simulink model "Scissor_Lift_4_Hydraulic_Actuator"  (R2016a)
settings: Solver=ode23t  StartTime=0.0  StopTime=10.0  MaxStep=1e-2  RelTol=1e-3  AbsTol=1e-4
PostLoadFcn:
  | warning off Simulink:Engine:OutputNotConnected
  | warning off mech2:compiler:topologyAnalysis:DanglingBlock
undefined symbols (not defined in the file): Local, Scissor_Lift_Param, X, Y, Z
libraries: sm_lib x48, Scissor_Parts_Lib x21, fl_lib x8, nesl_utility x7, sh_lib x4
(part 1 of 2)
Description:
  | Copyright 2014-2016 The MathWorks, Inc.
settings Model: Creator=smiller  LastModifiedBy=smiller
settings DataIOCC: LimitDataPoints=on  SaveFormat=Array  SignalLoggingSaveFormat=ModelDataLogs
settings OptimizationCC: ExpressionDepthLimit=2147483647
settings DebuggingCC: UnderspecifiedInitializationDetection=Classic  MergeDetectMultiDrivingBlocksExec=none  SolverPrmCheckMsg=warning  FcnCallInpInsideContextMsg=EnableAllAsWarning  AllowSymbolicDim=off  StateNameClashWarn=warning
settings HardwareCC: ProdBitPerPointer=32  ProdLargestAtomicFloat=None  ProdIntDivRoundTo=Undefined  ProdEndianess=Unspecified  ProdWordSize=32  ProdHWDeviceType=32-bit Generic
settings ModelReferenceCC: PropagateSignalLabelsOutOfModel=off
settings ConfigComp: CovModelRefEnable=Off  CovSFcnEnable=off
settings SimscapeCC: SimscapeLogType=all
settings ConfigurationSet: Description=SimMechanics 2G
settings ExplorerConfigSet: InternalSimMechanicsExplorerSettings="<ExplorerConfiguration><canonicalview>default</canonicalview><TilePanel><TileInfo><Tiles Columns=\"1\" Count=\"1\" Rows=\"1\"><Column Left=\"2\" Weight=\"1\"/><Column Left=\"398\"/><Row Top=\"2\" Weight=\"1\"/><Row Top=\"485\"/><Tile Height=\"1\" Width=\"1\" X=\"0\" Y=\"0\"/></Tiles></TileInfo><SceneInfo><SceneViewer><BGColor><R>0.60000002384185791</R><G>0.60000002384185791</G><B>0.60000002384185791</B></BGColor><Camera><Position><X>7.1151910018991291</X><Y>-6.9387533499588399</Y><Z>5.7460715877417217</Z></Position><Center><X>1.3999999761581421</X><Y>0</Y><Z>2.540661096572876</Z></Center><Up><X>-0.23055989473784222</X><Y>0.24511291789662082</Y><Z>0.94168030266045166</Z></Up><Left>-1.6691677093505861</Left><Right>1.6691677093505861</Right><Bottom>-3.5760457992553714</Bottom><Top>3.5760457992553714</Top></Camera></SceneViewer></SceneInfo></TilePanel></ExplorerConfiguration>"

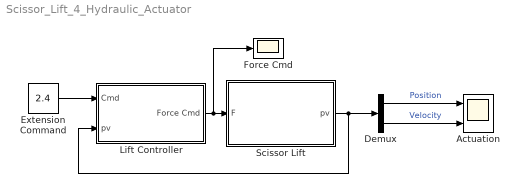
== system Scissor_Lift_4_Hydraulic_Actuator ==
  Actuation : Scope  NumInputPorts=2
  Demux : Demux  Outputs=2
  Extension Command : Constant  Value=2.4
  Force Cmd : Scope
  Lift Controller : Subsystem
  Scissor Lift : Subsystem
      mask Display:
      | image(imread('Scissor_Lift_3Stage_IMAGE.jpg'));
      | port_label('input',1,'F');
      | port_label('output',1,'pv');
  wires:
  Extension Command/1 -> Lift Controller/1(Cmd)
  Lift Controller/1(Force Cmd) -> Scissor Lift/1(F), Force Cmd/1
  Scissor Lift/1(pv) -> Lift Controller/2(pv), Demux/1
  Demux/1 -> Actuation/1  "Position"
  Demux/2 -> Actuation/2  "Velocity"

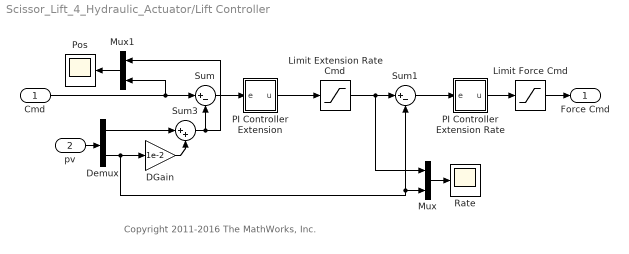
== system Scissor_Lift_4_Hydraulic_Actuator/Lift Controller ==
  note: Copyright 2011-2016 The MathWorks, Inc.
  Cmd : Inport
  pv : Inport  Port=2
  DGain : Gain  Gain=1e-2
  Demux : Demux  Outputs=2
  Limit Extension Rate Cmd : Saturate
  Limit Force Cmd : Saturate  UpperLimit=1e6  LowerLimit=-1e6
  Mux : Mux  Inputs=2
  Mux1 : Mux  Inputs=2
  PI Controller Extension : Subsystem
      mask Display:
      | plot([0 1],[0 0]);
      | plot([1 2],[0 1]);
      | plot([2 3],[1 1]);
      | disp('P I');
  PI Controller Extension Rate : Subsystem
      mask Display:
      | plot([0 1],[0 0]);
      | plot([1 2],[0 1]);
      | plot([2 3],[1 1]);
      | disp('P I');
  Pos : Scope
  Rate : Scope
  Sum : Sum  Inputs=|+-
  Sum1 : Sum  Inputs=|+-
  Sum3 : Sum  Inputs=|++
  Force Cmd : Outport
  wires:
  PI Controller Extension Rate/1(u) -> Limit Force Cmd/1
  PI Controller Extension/1(u) -> Limit Extension Rate Cmd/1
  Sum1/1 -> PI Controller Extension Rate/1(e)
  Limit Extension Rate Cmd/1 -> Sum1/1, Mux/1
  DGain/1 -> Sum3/2
  Sum3/1 -> Sum/2, Mux1/1
  Cmd/1 -> Sum/1, Mux1/2
  Sum/1 -> PI Controller Extension/1(e)
  Demux/2 -> DGain/1, Sum1/2, Mux/2
  Limit Force Cmd/1 -> Force Cmd/1
  Demux/1 -> Sum3/1
  pv/1 -> Demux/1
  Mux/1 -> Rate/1
  Mux1/1 -> Pos/1

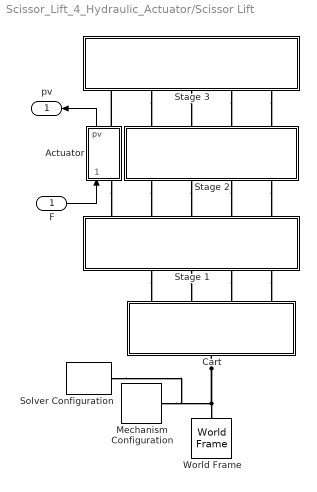
== system Scissor_Lift_4_Hydraulic_Actuator/Scissor Lift ==
  F : Inport
  Actuator : Subsystem
  Cart : Subsystem
  Mechanism Configuration : sm_lib/Utilities/Mechanism Configuration  UniformGravity=Constant  GravityVector=[0 0 -9.81]  GravityUnits=m/s^2  LinearizationDelta=0.001
  Solver Configuration : nesl_utility/Solver Configuration  PhysicalDomain=network_engine_domain  SubClassName=solver  LeftPortType=input  RightPortType=generic  Accelerate=off  Tones=[]  Harmonics=[]  SimulateNoise=off  Profile=off  UseLocalSampling=off  EnableSwitchedLinearOptims=on  FrequencyDomain=off  UseCCode=off  RelTol=0.001  AbsTol=1e-06  MinStep=1e-09  ToWorkspace=off  RevertToSquareIcSolve=off  NumHomotopyIterations=100  PhasorMode=off  PhasorModeNumHarmonics=1  OverrideAbsTol=off  DoDC=off  ResidualTolerance=1e-9  UseLocalSolver=off  LocalSolverChoice=NE_BACKWARD_EULER_ADVANCER  LocalSolverSampleTime=.001  DoFixedCost=off  MaxNonlinIter=3  MaxModeIter=2  LinearAlgebra=Sparse  DelaysMemoryBudget=1024  AutomaticFiltering=on  FilteringTimeConstant=0.001
  Stage 1 : Subsystem
  Stage 2 : Subsystem
  Stage 3 : Subsystem
  World Frame : sm_lib/Frames and Transforms/World Frame
  pv : Outport
  wires:
  Actuator/1(pv) -> pv/1
  F/1 -> Actuator/1(Vsig)
  connections:
  Actuator/LConn1 -- Stage 1/LConn1
  Actuator/RConn1 -- Stage 3/RConn1
  Cart/LConn1 -- Mechanism Configuration/RConn1 -- Solver Configuration/RConn1 -- World Frame/RConn1
  Stage 1/RConn2 -- Cart/RConn1
  Stage 1/RConn3 -- Cart/RConn2
  Stage 1/RConn4 -- Cart/RConn3
  Stage 1/RConn5 -- Cart/RConn4
  Stage 2/RConn1 -- Stage 1/LConn2
  Stage 2/RConn2 -- Stage 1/LConn3
  Stage 2/RConn3 -- Stage 1/LConn4
  Stage 2/RConn4 -- Stage 1/LConn5
  Stage 3/RConn2 -- Stage 2/LConn1
  Stage 3/RConn3 -- Stage 2/LConn2
  Stage 3/RConn4 -- Stage 2/LConn3
  Stage 3/RConn5 -- Stage 2/LConn4

== system Scissor_Lift_4_Hydraulic_Actuator/Lift Controller/PI Controller Extension ==
  e : Inport
  Integral Gain : Gain  Gain=100  SaturateOnIntegerOverflow=on  OutDataTypeStr=Inherit: Same as input  ParamDataTypeStr=Inherit: Same as input
  Integrator : Integrator  LimitOutput=on  UpperSaturationLimit=1  LowerSaturationLimit=-1
  Proportional Gain : Gain  Gain=8e2  SaturateOnIntegerOverflow=on  OutDataTypeStr=Inherit: Same as input  ParamDataTypeStr=Inherit: Same as input
  Sum : Sum  Inputs=++|  SaturateOnIntegerOverflow=on  InputSameDT=on  OutDataTypeStr=Inherit: Same as first input
  u : Outport  InitialOutput=0
  wires:
  Sum/1 -> u/1
  e/1 -> Integral Gain/1, Proportional Gain/1
  Integrator/1 -> Sum/2
  Proportional Gain/1 -> Sum/1
  Integral Gain/1 -> Integrator/1

== system Scissor_Lift_4_Hydraulic_Actuator/Lift Controller/PI Controller Extension Rate ==
  e : Inport
  Integral Gain : Gain  Gain=100  SaturateOnIntegerOverflow=on  OutDataTypeStr=Inherit: Same as input  ParamDataTypeStr=Inherit: Same as input
  Integrator : Integrator  LimitOutput=on  UpperSaturationLimit=1e6  LowerSaturationLimit=-1e6
  Proportional Gain : Gain  Gain=3e6  SaturateOnIntegerOverflow=on  OutDataTypeStr=Inherit: Same as input  ParamDataTypeStr=Inherit: Same as input
  Sum : Sum  Inputs=++|  SaturateOnIntegerOverflow=on  InputSameDT=on  OutDataTypeStr=Inherit: Same as first input
  u : Outport  InitialOutput=0
  wires:
  Integral Gain/1 -> Integrator/1
  Proportional Gain/1 -> Sum/1
  Integrator/1 -> Sum/2
  e/1 -> Proportional Gain/1, Integral Gain/1
  Sum/1 -> u/1

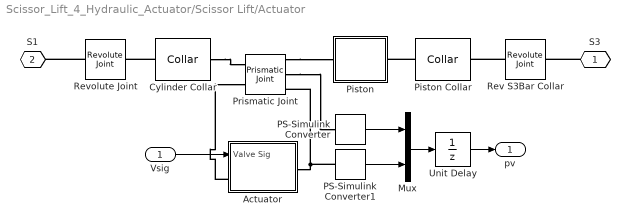
== system Scissor_Lift_4_Hydraulic_Actuator/Scissor Lift/Actuator ==
  Vsig : Inport
  Actuator : Subsystem
  Cylinder Collar : Scissor_Parts_Lib/Collar  collar_length=Scissor_Lift_Param.Actuator.Collar.Length  collar_radius=Scissor_Lift_Param.Actuator.Collar.Radius  cylinder_length=Scissor_Lift_Param.Actuator.Cylinder.Length  cylinder_radius=Scissor_Lift_Param.Actuator.Cylinder.Radius  cylinder_ori=Local +Z  material_density=Scissor_Lift_Param.Actuator.Collar.Density  material_color=Scissor_Lift_Param.Actuator.Collar.Color  material_opacity=Scissor_Lift_Param.Actuator.Collar.Opacity
  Mux : Mux  Inputs=2
  PS-Simulink Converter : nesl_utility/PS-Simulink Converter  PhysicalDomain=network_engine_domain  SubClassName=ps_output  LeftPortType=input  RightPortType=output  PseudoPeriodic=off  Frequencies=[]  Unit=1  AffineConversion=off
  PS-Simulink Converter1 : nesl_utility/PS-Simulink Converter  PhysicalDomain=network_engine_domain  SubClassName=ps_output  LeftPortType=input  RightPortType=output  PseudoPeriodic=off  Frequencies=[]  Unit=1  AffineConversion=off
  Piston : Subsystem
      mask Display:
      | image(imread('Piston_Shaft_IMAGE.jpg'));
      | port_label('RConn',1,'P');
      | port_label('LConn',1,'R');
  Piston Collar : Scissor_Parts_Lib/Collar  collar_length=Scissor_Lift_Param.Actuator.Collar.Length  collar_radius=Scissor_Lift_Param.Actuator.Collar.Radius  cylinder_length=Scissor_Lift_Param.Actuator.Piston_Seat.Length  cylinder_radius=Scissor_Lift_Param.Actuator.Piston_Seat.Radius  cylinder_ori=Local -Z  material_density=Scissor_Lift_Param.Actuator.Collar.Density  material_color=Scissor_Lift_Param.Actuator.Collar.Color  material_opacity=Scissor_Lift_Param.Actuator.Collar.Opacity
  Prismatic Joint : sm_lib/Joints/Prismatic Joint  SenseConstraintForce=off  SenseConstraintForceX=off  SenseConstraintForceY=off  SenseConstraintForceZ=off  SenseConstraintTorque=off  SenseConstraintTorqueX=off  SenseConstraintTorqueY=off  SenseConstraintTorqueZ=off  SenseTotalForce=off  SenseTotalForceX=off  SenseTotalForceY=off  SenseTotalForceZ=off  SenseTotalTorque=off  SenseTotalTorqueX=off  SenseTotalTorqueY=off  SenseTotalTorqueZ=off  CompositeWrenchDir=FollowerOnBase  CompositeWrenchFrame=BaseFrame  EquilibriumPosition=Scissor_Lift_Param.Actuator.Spring.Equilibrium_Position*0  EquilibriumPositionUnits=cm  SpringStiffness=Scissor_Lift_Param.Actuator.Spring.Stiffness*0  SpringStiffnessUnits=N/m  DampingCoefficient=Scissor_Lift_Param.Actuator.Spring.Damping*0+2000  DampingCoefficientUnits=N/(m/s)  TorqueActuationMode=InputTorque  MotionActuationMode=ComputedMotion  SensePosition=on  SenseVelocity=on  SenseAcceleration=off  SenseTorqueForce=off  PositionTargetSpecify=off  PositionTargetPriority=High  PositionTargetValue=0  PositionTargetValueUnits=m  VelocityTargetSpecify=off  VelocityTargetPriority=High  VelocityTargetValue=0  VelocityTargetValueUnits=m/s
  Rev S3Bar Collar : sm_lib/Joints/Revolute Joint  SenseConstraintForce=off  SenseConstraintForceX=off  SenseConstraintForceY=off  SenseConstraintForceZ=off  SenseConstraintTorque=off  SenseConstraintTorqueX=off  SenseConstraintTorqueY=off  SenseConstraintTorqueZ=off  SenseTotalForce=off  SenseTotalForceX=off  SenseTotalForceY=off  SenseTotalForceZ=off  SenseTotalTorque=off  SenseTotalTorqueX=off  SenseTotalTorqueY=off  SenseTotalTorqueZ=off  CompositeWrenchDir=FollowerOnBase  CompositeWrenchFrame=BaseFrame  EquilibriumPosition=0  EquilibriumPositionUnits=rad  SpringStiffness=0  SpringStiffnessUnits=N*m/rad  DampingCoefficient=0  DampingCoefficientUnits=N*m/(rad/s)  TorqueActuationMode=NoTorque  MotionActuationMode=ComputedMotion  SensePosition=off  SenseVelocity=off  SenseAcceleration=off  SenseTorqueForce=off  PositionTargetSpecify=off  PositionTargetPriority=High  PositionTargetValue=0  PositionTargetValueUnits=rad  VelocityTargetSpecify=off  VelocityTargetPriority=High  VelocityTargetValue=0  VelocityTargetValueUnits=rad/s
  Revolute Joint : sm_lib/Joints/Revolute Joint  SenseConstraintForce=off  SenseConstraintForceX=off  SenseConstraintForceY=off  SenseConstraintForceZ=off  SenseConstraintTorque=off  SenseConstraintTorqueX=off  SenseConstraintTorqueY=off  SenseConstraintTorqueZ=off  SenseTotalForce=off  SenseTotalForceX=off  SenseTotalForceY=off  SenseTotalForceZ=off  SenseTotalTorque=off  SenseTotalTorqueX=off  SenseTotalTorqueY=off  SenseTotalTorqueZ=off  CompositeWrenchDir=FollowerOnBase  CompositeWrenchFrame=BaseFrame  EquilibriumPosition=0  EquilibriumPositionUnits=rad  SpringStiffness=0  SpringStiffnessUnits=N*m/rad  DampingCoefficient=0  DampingCoefficientUnits=N*m/(rad/s)  TorqueActuationMode=NoTorque  MotionActuationMode=ComputedMotion  SensePosition=off  SenseVelocity=off  SenseAcceleration=off  SenseTorqueForce=off  PositionTargetSpecify=off  PositionTargetPriority=High  PositionTargetValue=0  PositionTargetValueUnits=rad  VelocityTargetSpecify=off  VelocityTargetPriority=High  VelocityTargetValue=0  VelocityTargetValueUnits=rad/s
  Unit Delay : UnitDelay  InitialCondition=1.755  SampleTime=0.01
  S3 : PMIOPort  Port=1  Side=Right
  S1 : PMIOPort  Port=2  Side=Left
  pv : Outport
  wires:
  Vsig/1 -> Actuator/1(Valve Sig)
  PS-Simulink Converter/1 -> Mux/1
  PS-Simulink Converter1/1 -> Mux/2
  Mux/1 -> Unit Delay/1
  Unit Delay/1 -> pv/1
  connections:
  Cylinder Collar/LConn1 -- Revolute Joint/RConn1
  Cylinder Collar/RConn1 -- Prismatic Joint/LConn1
  Prismatic Joint/RConn1 -- Piston/RConn1
  Piston Collar/RConn1 -- Piston/LConn1
  Rev S3Bar Collar/RConn1 -- Piston Collar/LConn1
  S3/RConn1 -- Rev S3Bar Collar/LConn1
  Revolute Joint/LConn1 -- S1/RConn1
  Prismatic Joint/RConn2 -- PS-Simulink Converter/LConn1
  Actuator/LConn1 -- Prismatic Joint/LConn2
  PS-Simulink Converter1/LConn1 -- Prismatic Joint/RConn3 -- Actuator/RConn1

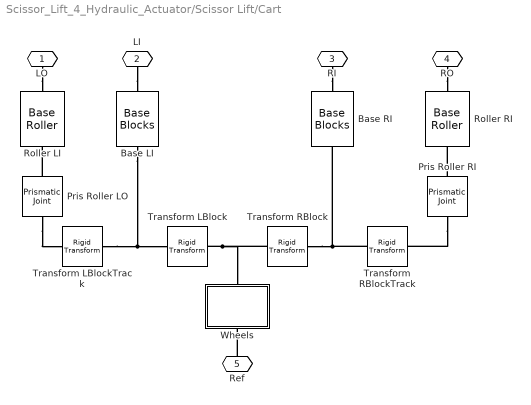
== system Scissor_Lift_4_Hydraulic_Actuator/Scissor Lift/Cart ==
  Base LI : Scissor_Parts_Lib/Base Blocks  block_length=Scissor_Lift_Param.Base_Block.Length  block_width=Scissor_Lift_Param.Base_Block.Width  block_height=Scissor_Lift_Param.Base_Block.Height  shaft_radius=Scissor_Lift_Param.Roller.Shaft_Radius  shaft_length=Scissor_Lift_Param.Roller.Shaft_Length  material_density=Scissor_Lift_Param.Base_Block.Density  material_color=Scissor_Lift_Param.Base_Block.Color  material_opacity=Scissor_Lift_Param.Base_Block.Opacity
  Base RI : Scissor_Parts_Lib/Base Blocks  block_length=Scissor_Lift_Param.Base_Block.Length  block_width=Scissor_Lift_Param.Base_Block.Width  block_height=Scissor_Lift_Param.Base_Block.Height  shaft_radius=Scissor_Lift_Param.Roller.Shaft_Radius  shaft_length=Scissor_Lift_Param.Roller.Shaft_Length  material_density=Scissor_Lift_Param.Base_Block.Density  material_color=Scissor_Lift_Param.Base_Block.Color  material_opacity=Scissor_Lift_Param.Base_Block.Opacity
  Pris Roller LO : sm_lib/Joints/Prismatic Joint  SenseConstraintForce=off  SenseConstraintForceX=off  SenseConstraintForceY=off  SenseConstraintForceZ=off  SenseConstraintTorque=off  SenseConstraintTorqueX=off  SenseConstraintTorqueY=off  SenseConstraintTorqueZ=off  SenseTotalForce=off  SenseTotalForceX=off  SenseTotalForceY=off  SenseTotalForceZ=off  SenseTotalTorque=off  SenseTotalTorqueX=off  SenseTotalTorqueY=off  SenseTotalTorqueZ=off  CompositeWrenchDir=FollowerOnBase  CompositeWrenchFrame=BaseFrame  EquilibriumPosition=0  EquilibriumPositionUnits=m  SpringStiffness=0  SpringStiffnessUnits=N/m  DampingCoefficient=0  DampingCoefficientUnits=N/(m/s)  TorqueActuationMode=NoTorque  MotionActuationMode=ComputedMotion  SensePosition=off  SenseVelocity=off  SenseAcceleration=off  SenseTorqueForce=off  PositionTargetSpecify=on  PositionTargetPriority=High  PositionTargetValue=Scissor_Lift_Param.Roller.Init_Pos_Target  PositionTargetValueUnits=cm  VelocityTargetSpecify=off  VelocityTargetPriority=High  VelocityTargetValue=0  VelocityTargetValueUnits=m/s
  Pris Roller RI : sm_lib/Joints/Prismatic Joint  SenseConstraintForce=off  SenseConstraintForceX=off  SenseConstraintForceY=off  SenseConstraintForceZ=off  SenseConstraintTorque=off  SenseConstraintTorqueX=off  SenseConstraintTorqueY=off  SenseConstraintTorqueZ=off  SenseTotalForce=off  SenseTotalForceX=off  SenseTotalForceY=off  SenseTotalForceZ=off  SenseTotalTorque=off  SenseTotalTorqueX=off  SenseTotalTorqueY=off  SenseTotalTorqueZ=off  CompositeWrenchDir=FollowerOnBase  CompositeWrenchFrame=BaseFrame  EquilibriumPosition=0  EquilibriumPositionUnits=m  SpringStiffness=0  SpringStiffnessUnits=N/m  DampingCoefficient=0  DampingCoefficientUnits=N/(m/s)  TorqueActuationMode=NoTorque  MotionActuationMode=ComputedMotion  SensePosition=off  SenseVelocity=off  SenseAcceleration=off  SenseTorqueForce=off  PositionTargetSpecify=off  PositionTargetPriority=High  PositionTargetValue=0  PositionTargetValueUnits=m  VelocityTargetSpecify=off  VelocityTargetPriority=High  VelocityTargetValue=0  VelocityTargetValueUnits=m/s
  Roller LI : Scissor_Parts_Lib/Base Roller  roller_length=Scissor_Lift_Param.Roller.Roller_Length  roller_radius=Scissor_Lift_Param.Roller.Roller_Radius  shaft_length=Scissor_Lift_Param.Roller.Shaft_Length  shaft_radius=Scissor_Lift_Param.Roller.Shaft_Radius  material_density=Scissor_Lift_Param.Roller.Density  material_color=Scissor_Lift_Param.Roller.Color  material_opacity=Scissor_Lift_Param.Roller.Opacity
  Roller RI : Scissor_Parts_Lib/Base Roller  roller_length=Scissor_Lift_Param.Roller.Roller_Length  roller_radius=Scissor_Lift_Param.Roller.Roller_Radius  shaft_length=Scissor_Lift_Param.Roller.Shaft_Length  shaft_radius=Scissor_Lift_Param.Roller.Shaft_Radius  material_density=Scissor_Lift_Param.Roller.Density  material_color=Scissor_Lift_Param.Roller.Color  material_opacity=Scissor_Lift_Param.Roller.Opacity
  Transform LBlock : sm_lib/Frames and Transforms/Rigid Transform  TranslationMethod=Cartesian  TranslationLengthUnit=cm  TranslationStandardAxis=+Y  TranslationStandardOffset=Scissor_Lift_Param.Cart.Platform.Height/2  TranslationCartesianOffset=[20 0 Scissor_Lift_Param.Link_Separation.Outer_Outer/2-Scissor_Lift_Param.Link_Separation.Outer_Inner]  TranslationROffset=0  TranslationROffsetUnits=m  TranslationZOffset=0  TranslationZOffsetUnits=m  TranslationThetaOffset=0  TranslationThetaOffsetUnits=deg  RotationMethod=None  RotationAngleUnits=deg  RotationStandardAxis=+X  RotationAngle=90  RotationArbitraryAxis=[0 0 1]  FollAlignAxisA=+X  BaseAlignAxisA=+Y  FollAlignAxisB=+Y  BaseAlignAxisB=+Z  RotationSequenceAxes=FollowerAxes  RotationSequence=XYX  RotationSequenceAngles=[0 0 0]  RotationSequenceAnglesUnits=deg  RotationMatrix=[1 0 0; 0 1 0; 0 0 1]
  Transform LBlockTrack : sm_lib/Frames and Transforms/Rigid Transform  TranslationMethod=StandardAxis  TranslationLengthUnit=cm  TranslationStandardAxis=+Z  TranslationStandardOffset=Scissor_Lift_Param.Link_Separation.Outer_Inner  TranslationCartesianOffset=[0 0 0]  TranslationROffset=0  TranslationROffsetUnits=m  TranslationZOffset=0  TranslationZOffsetUnits=m  TranslationThetaOffset=0  TranslationThetaOffsetUnits=deg  RotationMethod=StandardAxis  RotationAngleUnits=deg  RotationStandardAxis=+Y  RotationAngle=90  RotationArbitraryAxis=[0 0 1]  FollAlignAxisA=+X  BaseAlignAxisA=+Y  FollAlignAxisB=+Y  BaseAlignAxisB=+Z  RotationSequenceAxes=FollowerAxes  RotationSequence=XYX  RotationSequenceAngles=[0 0 0]  RotationSequenceAnglesUnits=deg  RotationMatrix=[1 0 0; 0 1 0; 0 0 1]
  Transform RBlock : sm_lib/Frames and Transforms/Rigid Transform  TranslationMethod=Cartesian  TranslationLengthUnit=cm  TranslationStandardAxis=+Y  TranslationStandardOffset=Scissor_Lift_Param.Cart.Platform.Height/2  TranslationCartesianOffset=[20 0 -Scissor_Lift_Param.Link_Separation.Outer_Outer/2+Scissor_Lift_Param.Link_Separation.Outer_Inner]  TranslationROffset=0  TranslationROffsetUnits=m  TranslationZOffset=0  TranslationZOffsetUnits=m  TranslationThetaOffset=0  TranslationThetaOffsetUnits=deg  RotationMethod=None  RotationAngleUnits=deg  RotationStandardAxis=+X  RotationAngle=90  RotationArbitraryAxis=[0 0 1]  FollAlignAxisA=+X  BaseAlignAxisA=+Y  FollAlignAxisB=+Y  BaseAlignAxisB=+Z  RotationSequenceAxes=FollowerAxes  RotationSequence=XYX  RotationSequenceAngles=[0 0 0]  RotationSequenceAnglesUnits=deg  RotationMatrix=[1 0 0; 0 1 0; 0 0 1]
  Transform RBlockTrack : sm_lib/Frames and Transforms/Rigid Transform  TranslationMethod=StandardAxis  TranslationLengthUnit=cm  TranslationStandardAxis=-Z  TranslationStandardOffset=Scissor_Lift_Param.Link_Separation.Outer_Inner  TranslationCartesianOffset=[0 0 0]  TranslationROffset=0  TranslationROffsetUnits=m  TranslationZOffset=0  TranslationZOffsetUnits=m  TranslationThetaOffset=0  TranslationThetaOffsetUnits=deg  RotationMethod=StandardAxis  RotationAngleUnits=deg  RotationStandardAxis=+Y  RotationAngle=90  RotationArbitraryAxis=[0 0 1]  FollAlignAxisA=+X  BaseAlignAxisA=+Y  FollAlignAxisB=+Y  BaseAlignAxisB=+Z  RotationSequenceAxes=FollowerAxes  RotationSequence=XYX  RotationSequenceAngles=[0 0 0]  RotationSequenceAnglesUnits=deg  RotationMatrix=[1 0 0; 0 1 0; 0 0 1]
  Wheels : Subsystem
  LO : PMIOPort  Port=1  Side=Right
  LI : PMIOPort  Port=2  Side=Right
  RI : PMIOPort  Port=3  Side=Right
  RO : PMIOPort  Port=4  Side=Right
  Ref : PMIOPort  Port=5  Side=Left
  connections:
  Pris Roller LO/LConn1 -- Transform LBlockTrack/RConn1
  Pris Roller LO/RConn1 -- Roller LI/LConn1
  Transform LBlockTrack/LConn1 -- Base LI/LConn1 -- Transform LBlock/RConn1
  Transform RBlockTrack/LConn1 -- Base RI/LConn1 -- Transform RBlock/RConn1
  Pris Roller RI/LConn1 -- Transform RBlockTrack/RConn1
  Pris Roller RI/RConn1 -- Roller RI/LConn1
  Ref/RConn1 -- Wheels/LConn1
  LO/RConn1 -- Roller LI/RConn1
  LI/RConn1 -- Base LI/RConn1
  RO/RConn1 -- Roller RI/RConn1
  RI/RConn1 -- Base RI/RConn1
  Transform LBlock/LConn1 -- Wheels/RConn1 -- Transform RBlock/LConn1

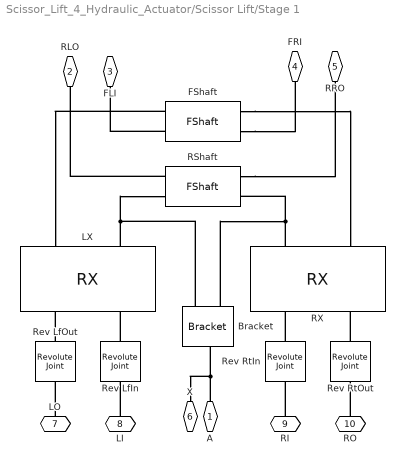
== system Scissor_Lift_4_Hydraulic_Actuator/Scissor Lift/Stage 1 ==
  Bracket : Scissor_Parts_Lib/Bracket  fl_w=Scissor_Lift_Param.Actuator.Bracket.Flange.Width  fl_h=Scissor_Lift_Param.Actuator.Bracket.Flange.Height  T=Scissor_Lift_Param.Actuator.Bracket.Flange.Thickness  W=Scissor_Lift_Param.Actuator.Bracket.Flange.Offset  flupdown=Down  flfrontrear=Rear  fl_density=Scissor_Lift_Param.Actuator.Bracket.Flange.Density  fl_clr=Scissor_Lift_Param.Actuator.Bracket.Flange.Color  fl_opc=Scissor_Lift_Param.Actuator.Bracket.Flange.Opacity  shaft_length=Scissor_Lift_Param.Link_Separation.Outer_Outer-Scissor_Lift_Param.Link_Separation.Outer_Inner*2  shaft_radius=Scissor_Lift_Param.Actuator.Bracket.Shaft.Radius  shaft_density=Scissor_Lift_Param.Actuator.Bracket.Shaft.Density  shaft_color=Scissor_Lift_Param.Actuator.Bracket.Shaft.Color  shaft_opacity=Scissor_Lift_Param.Actuator.Bracket.Shaft.Opacity
  FShaft : Scissor_Parts_Lib/FShaft  sep_outer_outer=Scissor_Lift_Param.Link_Separation.Outer_Outer  sep_outer_inner=Scissor_Lift_Param.Link_Separation.Outer_Inner  shaft_radius=Scissor_Lift_Param.Trans_Shaft.Radius  shaft_density=Scissor_Lift_Param.Trans_Shaft.Density  shaft_color=Scissor_Lift_Param.Trans_Shaft.Color  shaft_opacity=Scissor_Lift_Param.Trans_Shaft.Opacity
  LX : Scissor_Parts_Lib/RX  link_length=Scissor_Lift_Param.Link.Length  link_width=Scissor_Lift_Param.Link.Width  link_thickness=Scissor_Lift_Param.Link.Thickness  link_hole_radius=Scissor_Lift_Param.Link.Hole_Radius  link_density=Scissor_Lift_Param.Link.Density  link_color=Scissor_Lift_Param.Link.Color  link_opacity=Scissor_Lift_Param.Link.Opacity  shaft_length=Scissor_Lift_Param.Link_Separation.Outer_Inner  shaft_radius=Scissor_Lift_Param.Link_Pin.Radius  shaft_density=Scissor_Lift_Param.Link_Pin.Density  shaft_color=Scissor_Lift_Param.Link_Pin.Color  shaft_opacity=Scissor_Lift_Param.Link_Pin.Opacity  leftright=Left  imgfile=Crossbar_RX_IMAGE.jpg  L1Port=OU  L2Port=IU  R1Port=OL  R2Port=IL
  RShaft : Scissor_Parts_Lib/FShaft  sep_outer_outer=Scissor_Lift_Param.Link_Separation.Outer_Outer  sep_outer_inner=Scissor_Lift_Param.Link_Separation.Outer_Inner  shaft_radius=Scissor_Lift_Param.Trans_Shaft.Radius  shaft_density=Scissor_Lift_Param.Trans_Shaft.Density  shaft_color=Scissor_Lift_Param.Trans_Shaft.Color  shaft_opacity=Scissor_Lift_Param.Trans_Shaft.Opacity
  RX : Scissor_Parts_Lib/RX  link_length=Scissor_Lift_Param.Link.Length  link_width=Scissor_Lift_Param.Link.Width  link_thickness=Scissor_Lift_Param.Link.Thickness  link_hole_radius=Scissor_Lift_Param.Link.Hole_Radius  link_density=Scissor_Lift_Param.Link.Density  link_color=Scissor_Lift_Param.Link.Color  link_opacity=Scissor_Lift_Param.Link.Opacity  shaft_length=Scissor_Lift_Param.Link_Separation.Outer_Inner  shaft_radius=Scissor_Lift_Param.Link_Pin.Radius  shaft_density=Scissor_Lift_Param.Link_Pin.Density  shaft_color=Scissor_Lift_Param.Link_Pin.Color  shaft_opacity=Scissor_Lift_Param.Link_Pin.Opacity  leftright=Right  imgfile=Crossbar_RX_IMAGE.jpg  L1Port=OU  L2Port=IU  R1Port=OL  R2Port=IL
  Rev LfIn : sm_lib/Joints/Revolute Joint  SenseConstraintForce=off  SenseConstraintForceX=off  SenseConstraintForceY=off  SenseConstraintForceZ=off  SenseConstraintTorque=off  SenseConstraintTorqueX=off  SenseConstraintTorqueY=off  SenseConstraintTorqueZ=off  SenseTotalForce=off  SenseTotalForceX=off  SenseTotalForceY=off  SenseTotalForceZ=off  SenseTotalTorque=off  SenseTotalTorqueX=off  SenseTotalTorqueY=off  SenseTotalTorqueZ=off  CompositeWrenchDir=FollowerOnBase  CompositeWrenchFrame=BaseFrame  EquilibriumPosition=0  EquilibriumPositionUnits=rad  SpringStiffness=0  SpringStiffnessUnits=N*m/rad  DampingCoefficient=0  DampingCoefficientUnits=N*m/(rad/s)  TorqueActuationMode=NoTorque  MotionActuationMode=ComputedMotion  SensePosition=off  SenseVelocity=off  SenseAcceleration=off  SenseTorqueForce=off  PositionTargetSpecify=off  PositionTargetPriority=Low  PositionTargetValue=0  PositionTargetValueUnits=deg  VelocityTargetSpecify=off  VelocityTargetPriority=High  VelocityTargetValue=0  VelocityTargetValueUnits=rad/s
  Rev LfOut : sm_lib/Joints/Revolute Joint  SenseConstraintForce=off  SenseConstraintForceX=off  SenseConstraintForceY=off  SenseConstraintForceZ=off  SenseConstraintTorque=off  SenseConstraintTorqueX=off  SenseConstraintTorqueY=off  SenseConstraintTorqueZ=off  SenseTotalForce=off  SenseTotalForceX=off  SenseTotalForceY=off  SenseTotalForceZ=off  SenseTotalTorque=off  SenseTotalTorqueX=off  SenseTotalTorqueY=off  SenseTotalTorqueZ=off  CompositeWrenchDir=FollowerOnBase  CompositeWrenchFrame=BaseFrame  EquilibriumPosition=0  EquilibriumPositionUnits=rad  SpringStiffness=0  SpringStiffnessUnits=N*m/rad  DampingCoefficient=0  DampingCoefficientUnits=N*m/(rad/s)  TorqueActuationMode=NoTorque  MotionActuationMode=ComputedMotion  SensePosition=off  SenseVelocity=off  SenseAcceleration=off  SenseTorqueForce=off  PositionTargetSpecify=on  PositionTargetPriority=Low  PositionTargetValue=Scissor_Lift_Param.Crossbar.Init_Angle_Target  PositionTargetValueUnits=deg  VelocityTargetSpecify=off  VelocityTargetPriority=High  VelocityTargetValue=0  VelocityTargetValueUnits=rad/s
  Rev RtIn : sm_lib/Joints/Revolute Joint  SenseConstraintForce=off  SenseConstraintForceX=off  SenseConstraintForceY=off  SenseConstraintForceZ=off  SenseConstraintTorque=off  SenseConstraintTorqueX=off  SenseConstraintTorqueY=off  SenseConstraintTorqueZ=off  SenseTotalForce=off  SenseTotalForceX=off  SenseTotalForceY=off  SenseTotalForceZ=off  SenseTotalTorque=off  SenseTotalTorqueX=off  SenseTotalTorqueY=off  SenseTotalTorqueZ=off  CompositeWrenchDir=FollowerOnBase  CompositeWrenchFrame=BaseFrame  EquilibriumPosition=0  EquilibriumPositionUnits=rad  SpringStiffness=0  SpringStiffnessUnits=N*m/rad  DampingCoefficient=0  DampingCoefficientUnits=N*m/(rad/s)  TorqueActuationMode=NoTorque  MotionActuationMode=ComputedMotion  SensePosition=off  SenseVelocity=off  SenseAcceleration=off  SenseTorqueForce=off  PositionTargetSpecify=off  PositionTargetPriority=Low  PositionTargetValue=0  PositionTargetValueUnits=deg  VelocityTargetSpecify=off  VelocityTargetPriority=High  VelocityTargetValue=0  VelocityTargetValueUnits=rad/s
  Rev RtOut : sm_lib/Joints/Revolute Joint  SenseConstraintForce=off  SenseConstraintForceX=off  SenseConstraintForceY=off  SenseConstraintForceZ=off  SenseConstraintTorque=off  SenseConstraintTorqueX=off  SenseConstraintTorqueY=off  SenseConstraintTorqueZ=off  SenseTotalForce=off  SenseTotalForceX=off  SenseTotalForceY=off  SenseTotalForceZ=off  SenseTotalTorque=off  SenseTotalTorqueX=off  SenseTotalTorqueY=off  SenseTotalTorqueZ=off  CompositeWrenchDir=FollowerOnBase  CompositeWrenchFrame=BaseFrame  EquilibriumPosition=0  EquilibriumPositionUnits=rad  SpringStiffness=0  SpringStiffnessUnits=N*m/rad  DampingCoefficient=0  DampingCoefficientUnits=N*m/(rad/s)  TorqueActuationMode=NoTorque  MotionActuationMode=ComputedMotion  SensePosition=off  SenseVelocity=off  SenseAcceleration=off  SenseTorqueForce=off  PositionTargetSpecify=off  PositionTargetPriority=Low  PositionTargetValue=0  PositionTargetValueUnits=deg  VelocityTargetSpecify=off  VelocityTargetPriority=High  VelocityTargetValue=0  VelocityTargetValueUnits=rad/s
  A : PMIOPort  Port=1  Side=Left
  RLO : PMIOPort  Port=2  Side=Left
  FLI : PMIOPort  Port=3  Side=Left
  FRI : PMIOPort  Port=4  Side=Left
  RRO : PMIOPort  Port=5  Side=Left
  X : PMIOPort  Port=6  Side=Right
  LO : PMIOPort  Port=7  Side=Right
  LI : PMIOPort  Port=8  Side=Right
  RI : PMIOPort  Port=9  Side=Right
  RO : PMIOPort  Port=10  Side=Right
  connections:
  FShaft/LConn1 -- LX/LConn1
  FShaft/LConn2 -- FLI/RConn1
  FShaft/RConn1 -- RX/LConn2
  FShaft/RConn2 -- FRI/RConn1
  LX/LConn2 -- RShaft/LConn2 -- Bracket/RConn1
  Rev LfOut/RConn1 -- LX/RConn1
  Rev LfIn/RConn1 -- LX/RConn2
  RShaft/LConn1 -- RLO/RConn1
  RShaft/RConn1 -- RRO/RConn1
  RX/LConn1 -- RShaft/RConn2 -- Bracket/RConn2
  Rev RtIn/RConn1 -- RX/RConn1
  Rev RtOut/RConn1 -- RX/RConn2
  LI/RConn1 -- Rev LfIn/LConn1
  LO/RConn1 -- Rev LfOut/LConn1
  RI/RConn1 -- Rev RtIn/LConn1
  RO/RConn1 -- Rev RtOut/LConn1
  Bracket/LConn1 -- X/RConn1 -- A/RConn1

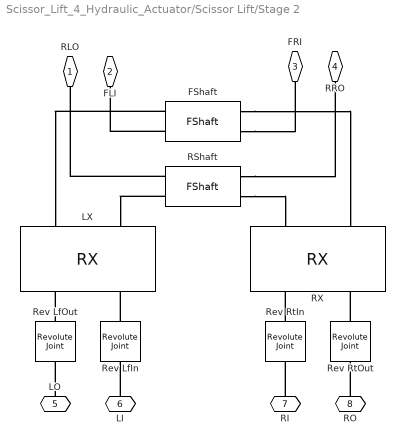
== system Scissor_Lift_4_Hydraulic_Actuator/Scissor Lift/Stage 2 ==
  FShaft : Scissor_Parts_Lib/FShaft  sep_outer_outer=Scissor_Lift_Param.Link_Separation.Outer_Outer  sep_outer_inner=Scissor_Lift_Param.Link_Separation.Outer_Inner  shaft_radius=Scissor_Lift_Param.Trans_Shaft.Radius  shaft_density=Scissor_Lift_Param.Trans_Shaft.Density  shaft_color=Scissor_Lift_Param.Trans_Shaft.Color  shaft_opacity=Scissor_Lift_Param.Trans_Shaft.Opacity
  LX : Scissor_Parts_Lib/RX  link_length=Scissor_Lift_Param.Link.Length  link_width=Scissor_Lift_Param.Link.Width  link_thickness=Scissor_Lift_Param.Link.Thickness  link_hole_radius=Scissor_Lift_Param.Link.Hole_Radius  link_density=Scissor_Lift_Param.Link.Density  link_color=Scissor_Lift_Param.Link.Color  link_opacity=Scissor_Lift_Param.Link.Opacity  shaft_length=Scissor_Lift_Param.Link_Separation.Outer_Inner  shaft_radius=Scissor_Lift_Param.Link_Pin.Radius  shaft_density=Scissor_Lift_Param.Link_Pin.Density  shaft_color=Scissor_Lift_Param.Link_Pin.Color  shaft_opacity=Scissor_Lift_Param.Link_Pin.Opacity  leftright=Left  imgfile=Crossbar_RX_IMAGE.jpg  L1Port=OU  L2Port=IU  R1Port=OL  R2Port=IL
  RShaft : Scissor_Parts_Lib/FShaft  sep_outer_outer=Scissor_Lift_Param.Link_Separation.Outer_Outer  sep_outer_inner=Scissor_Lift_Param.Link_Separation.Outer_Inner  shaft_radius=Scissor_Lift_Param.Trans_Shaft.Radius  shaft_density=Scissor_Lift_Param.Trans_Shaft.Density  shaft_color=Scissor_Lift_Param.Trans_Shaft.Color  shaft_opacity=Scissor_Lift_Param.Trans_Shaft.Opacity
  RX : Scissor_Parts_Lib/RX  link_length=Scissor_Lift_Param.Link.Length  link_width=Scissor_Lift_Param.Link.Width  link_thickness=Scissor_Lift_Param.Link.Thickness  link_hole_radius=Scissor_Lift_Param.Link.Hole_Radius  link_density=Scissor_Lift_Param.Link.Density  link_color=Scissor_Lift_Param.Link.Color  link_opacity=Scissor_Lift_Param.Link.Opacity  shaft_length=Scissor_Lift_Param.Link_Separation.Outer_Inner  shaft_radius=Scissor_Lift_Param.Link_Pin.Radius  shaft_density=Scissor_Lift_Param.Link_Pin.Density  shaft_color=Scissor_Lift_Param.Link_Pin.Color  shaft_opacity=Scissor_Lift_Param.Link_Pin.Opacity  leftright=Right  imgfile=Crossbar_RX_IMAGE.jpg  L1Port=OU  L2Port=IU  R1Port=OL  R2Port=IL
  Rev LfIn : sm_lib/Joints/Revolute Joint  SenseConstraintForce=off  SenseConstraintForceX=off  SenseConstraintForceY=off  SenseConstraintForceZ=off  SenseConstraintTorque=off  SenseConstraintTorqueX=off  SenseConstraintTorqueY=off  SenseConstraintTorqueZ=off  SenseTotalForce=off  SenseTotalForceX=off  SenseTotalForceY=off  SenseTotalForceZ=off  SenseTotalTorque=off  SenseTotalTorqueX=off  SenseTotalTorqueY=off  SenseTotalTorqueZ=off  CompositeWrenchDir=FollowerOnBase  CompositeWrenchFrame=BaseFrame  EquilibriumPosition=0  EquilibriumPositionUnits=rad  SpringStiffness=0  SpringStiffnessUnits=N*m/rad  DampingCoefficient=0  DampingCoefficientUnits=N*m/(rad/s)  TorqueActuationMode=NoTorque  MotionActuationMode=ComputedMotion  SensePosition=off  SenseVelocity=off  SenseAcceleration=off  SenseTorqueForce=off  PositionTargetSpecify=off  PositionTargetPriority=Low  PositionTargetValue=0  PositionTargetValueUnits=deg  VelocityTargetSpecify=off  VelocityTargetPriority=High  VelocityTargetValue=0  VelocityTargetValueUnits=rad/s
  Rev LfOut : sm_lib/Joints/Revolute Joint  SenseConstraintForce=off  SenseConstraintForceX=off  SenseConstraintForceY=off  SenseConstraintForceZ=off  SenseConstraintTorque=off  SenseConstraintTorqueX=off  SenseConstraintTorqueY=off  SenseConstraintTorqueZ=off  SenseTotalForce=off  SenseTotalForceX=off  SenseTotalForceY=off  SenseTotalForceZ=off  SenseTotalTorque=off  SenseTotalTorqueX=off  SenseTotalTorqueY=off  SenseTotalTorqueZ=off  CompositeWrenchDir=FollowerOnBase  CompositeWrenchFrame=BaseFrame  EquilibriumPosition=0  EquilibriumPositionUnits=rad  SpringStiffness=0  SpringStiffnessUnits=N*m/rad  DampingCoefficient=0  DampingCoefficientUnits=N*m/(rad/s)  TorqueActuationMode=NoTorque  MotionActuationMode=ComputedMotion  SensePosition=off  SenseVelocity=off  SenseAcceleration=off  SenseTorqueForce=off  PositionTargetSpecify=on  PositionTargetPriority=Low  PositionTargetValue=2*Scissor_Lift_Param.Crossbar.Init_Angle_Target  PositionTargetValueUnits=deg  VelocityTargetSpecify=off  VelocityTargetPriority=High  VelocityTargetValue=0  VelocityTargetValueUnits=rad/s
  Rev RtIn : sm_lib/Joints/Revolute Joint  SenseConstraintForce=off  SenseConstraintForceX=off  SenseConstraintForceY=off  SenseConstraintForceZ=off  SenseConstraintTorque=off  SenseConstraintTorqueX=off  SenseConstraintTorqueY=off  SenseConstraintTorqueZ=off  SenseTotalForce=off  SenseTotalForceX=off  SenseTotalForceY=off  SenseTotalForceZ=off  SenseTotalTorque=off  SenseTotalTorqueX=off  SenseTotalTorqueY=off  SenseTotalTorqueZ=off  CompositeWrenchDir=FollowerOnBase  CompositeWrenchFrame=BaseFrame  EquilibriumPosition=0  EquilibriumPositionUnits=rad  SpringStiffness=0  SpringStiffnessUnits=N*m/rad  DampingCoefficient=0  DampingCoefficientUnits=N*m/(rad/s)  TorqueActuationMode=NoTorque  MotionActuationMode=ComputedMotion  SensePosition=off  SenseVelocity=off  SenseAcceleration=off  SenseTorqueForce=off  PositionTargetSpecify=off  PositionTargetPriority=Low  PositionTargetValue=0  PositionTargetValueUnits=deg  VelocityTargetSpecify=off  VelocityTargetPriority=High  VelocityTargetValue=0  VelocityTargetValueUnits=rad/s
  Rev RtOut : sm_lib/Joints/Revolute Joint  SenseConstraintForce=off  SenseConstraintForceX=off  SenseConstraintForceY=off  SenseConstraintForceZ=off  SenseConstraintTorque=off  SenseConstraintTorqueX=off  SenseConstraintTorqueY=off  SenseConstraintTorqueZ=off  SenseTotalForce=off  SenseTotalForceX=off  SenseTotalForceY=off  SenseTotalForceZ=off  SenseTotalTorque=off  SenseTotalTorqueX=off  SenseTotalTorqueY=off  SenseTotalTorqueZ=off  CompositeWrenchDir=FollowerOnBase  CompositeWrenchFrame=BaseFrame  EquilibriumPosition=0  EquilibriumPositionUnits=rad  SpringStiffness=0  SpringStiffnessUnits=N*m/rad  DampingCoefficient=0  DampingCoefficientUnits=N*m/(rad/s)  TorqueActuationMode=NoTorque  MotionActuationMode=ComputedMotion  SensePosition=off  SenseVelocity=off  SenseAcceleration=off  SenseTorqueForce=off  PositionTargetSpecify=off  PositionTargetPriority=Low  PositionTargetValue=0  PositionTargetValueUnits=deg  VelocityTargetSpecify=off  VelocityTargetPriority=High  VelocityTargetValue=0  VelocityTargetValueUnits=rad/s
  RLO : PMIOPort  Port=1  Side=Left
  FLI : PMIOPort  Port=2  Side=Left
  FRI : PMIOPort  Port=3  Side=Left
  RRO : PMIOPort  Port=4  Side=Left
  LO : PMIOPort  Port=5  Side=Right
  LI : PMIOPort  Port=6  Side=Right
  RI : PMIOPort  Port=7  Side=Right
  RO : PMIOPort  Port=8  Side=Right
  connections:
  RO/RConn1 -- Rev RtOut/LConn1
  RI/RConn1 -- Rev RtIn/LConn1
  LO/RConn1 -- Rev LfOut/LConn1
  LI/RConn1 -- Rev LfIn/LConn1
  Rev RtOut/RConn1 -- RX/RConn2
  Rev RtIn/RConn1 -- RX/RConn1
  RShaft/RConn2 -- RX/LConn1
  RShaft/RConn1 -- RRO/RConn1
  RShaft/LConn1 -- RLO/RConn1
  Rev LfIn/RConn1 -- LX/RConn2
  Rev LfOut/RConn1 -- LX/RConn1
  RShaft/LConn2 -- LX/LConn2
  FShaft/RConn2 -- FRI/RConn1
  FShaft/RConn1 -- RX/LConn2
  FShaft/LConn2 -- FLI/RConn1
  FShaft/LConn1 -- LX/LConn1

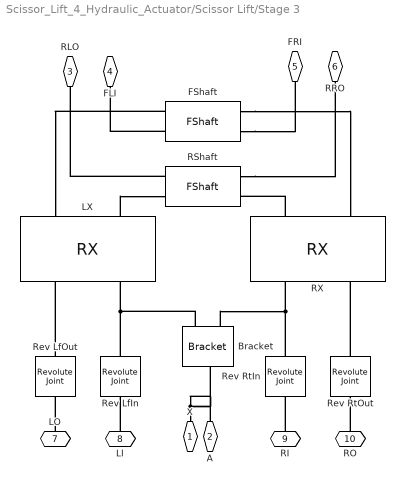
== system Scissor_Lift_4_Hydraulic_Actuator/Scissor Lift/Stage 3 ==
  Bracket : Scissor_Parts_Lib/Bracket  fl_w=Scissor_Lift_Param.Actuator.Bracket.Flange.Width  fl_h=Scissor_Lift_Param.Actuator.Bracket.Flange.Height  T=Scissor_Lift_Param.Actuator.Bracket.Flange.Thickness  W=Scissor_Lift_Param.Actuator.Bracket.Flange.Offset  flupdown=Up  flfrontrear=Front  fl_density=Scissor_Lift_Param.Actuator.Bracket.Flange.Density  fl_clr=Scissor_Lift_Param.Actuator.Bracket.Flange.Color  fl_opc=Scissor_Lift_Param.Actuator.Bracket.Flange.Opacity  shaft_length=Scissor_Lift_Param.Link_Separation.Outer_Outer-Scissor_Lift_Param.Link_Separation.Outer_Inner*2  shaft_radius=Scissor_Lift_Param.Actuator.Bracket.Shaft.Radius  shaft_density=Scissor_Lift_Param.Actuator.Bracket.Shaft.Density  shaft_color=Scissor_Lift_Param.Actuator.Bracket.Shaft.Color  shaft_opacity=Scissor_Lift_Param.Actuator.Bracket.Shaft.Opacity
  FShaft : Scissor_Parts_Lib/FShaft  sep_outer_outer=Scissor_Lift_Param.Link_Separation.Outer_Outer  sep_outer_inner=Scissor_Lift_Param.Link_Separation.Outer_Inner  shaft_radius=Scissor_Lift_Param.Trans_Shaft.Radius  shaft_density=Scissor_Lift_Param.Trans_Shaft.Density  shaft_color=Scissor_Lift_Param.Trans_Shaft.Color  shaft_opacity=Scissor_Lift_Param.Trans_Shaft.Opacity
  LX : Scissor_Parts_Lib/RX  link_length=Scissor_Lift_Param.Link.Length  link_width=Scissor_Lift_Param.Link.Width  link_thickness=Scissor_Lift_Param.Link.Thickness  link_hole_radius=Scissor_Lift_Param.Link.Hole_Radius  link_density=Scissor_Lift_Param.Link.Density  link_color=Scissor_Lift_Param.Link.Color  link_opacity=Scissor_Lift_Param.Link.Opacity  shaft_length=Scissor_Lift_Param.Link_Separation.Outer_Inner  shaft_radius=Scissor_Lift_Param.Link_Pin.Radius  shaft_density=Scissor_Lift_Param.Link_Pin.Density  shaft_color=Scissor_Lift_Param.Link_Pin.Color  shaft_opacity=Scissor_Lift_Param.Link_Pin.Opacity  leftright=Left  imgfile=Crossbar_RX_IMAGE.jpg  L1Port=OU  L2Port=IU  R1Port=OL  R2Port=IL
  RShaft : Scissor_Parts_Lib/FShaft  sep_outer_outer=Scissor_Lift_Param.Link_Separation.Outer_Outer  sep_outer_inner=Scissor_Lift_Param.Link_Separation.Outer_Inner  shaft_radius=Scissor_Lift_Param.Trans_Shaft.Radius  shaft_density=Scissor_Lift_Param.Trans_Shaft.Density  shaft_color=Scissor_Lift_Param.Trans_Shaft.Color  shaft_opacity=Scissor_Lift_Param.Trans_Shaft.Opacity
  RX : Scissor_Parts_Lib/RX  link_length=Scissor_Lift_Param.Link.Length  link_width=Scissor_Lift_Param.Link.Width  link_thickness=Scissor_Lift_Param.Link.Thickness  link_hole_radius=Scissor_Lift_Param.Link.Hole_Radius  link_density=Scissor_Lift_Param.Link.Density  link_color=Scissor_Lift_Param.Link.Color  link_opacity=Scissor_Lift_Param.Link.Opacity  shaft_length=Scissor_Lift_Param.Link_Separation.Outer_Inner  shaft_radius=Scissor_Lift_Param.Link_Pin.Radius  shaft_density=Scissor_Lift_Param.Link_Pin.Density  shaft_color=Scissor_Lift_Param.Link_Pin.Color  shaft_opacity=Scissor_Lift_Param.Link_Pin.Opacity  leftright=Right  imgfile=Crossbar_RX_IMAGE.jpg  L1Port=OU  L2Port=IU  R1Port=OL  R2Port=IL
  Rev LfIn : sm_lib/Joints/Revolute Joint  SenseConstraintForce=off  SenseConstraintForceX=off  SenseConstraintForceY=off  SenseConstraintForceZ=off  SenseConstraintTorque=off  SenseConstraintTorqueX=off  SenseConstraintTorqueY=off  SenseConstraintTorqueZ=off  SenseTotalForce=off  SenseTotalForceX=off  SenseTotalForceY=off  SenseTotalForceZ=off  SenseTotalTorque=off  SenseTotalTorqueX=off  SenseTotalTorqueY=off  SenseTotalTorqueZ=off  CompositeWrenchDir=FollowerOnBase  CompositeWrenchFrame=BaseFrame  EquilibriumPosition=0  EquilibriumPositionUnits=rad  SpringStiffness=0  SpringStiffnessUnits=N*m/rad  DampingCoefficient=0  DampingCoefficientUnits=N*m/(rad/s)  TorqueActuationMode=NoTorque  MotionActuationMode=ComputedMotion  SensePosition=off  SenseVelocity=off  SenseAcceleration=off  SenseTorqueForce=off  PositionTargetSpecify=off  PositionTargetPriority=Low  PositionTargetValue=0  PositionTargetValueUnits=deg  VelocityTargetSpecify=off  VelocityTargetPriority=High  VelocityTargetValue=0  VelocityTargetValueUnits=rad/s
  Rev LfOut : sm_lib/Joints/Revolute Joint  SenseConstraintForce=off  SenseConstraintForceX=off  SenseConstraintForceY=off  SenseConstraintForceZ=off  SenseConstraintTorque=off  SenseConstraintTorqueX=off  SenseConstraintTorqueY=off  SenseConstraintTorqueZ=off  SenseTotalForce=off  SenseTotalForceX=off  SenseTotalForceY=off  SenseTotalForceZ=off  SenseTotalTorque=off  SenseTotalTorqueX=off  SenseTotalTorqueY=off  SenseTotalTorqueZ=off  CompositeWrenchDir=FollowerOnBase  CompositeWrenchFrame=BaseFrame  EquilibriumPosition=0  EquilibriumPositionUnits=rad  SpringStiffness=0  SpringStiffnessUnits=N*m/rad  DampingCoefficient=0  DampingCoefficientUnits=N*m/(rad/s)  TorqueActuationMode=NoTorque  MotionActuationMode=ComputedMotion  SensePosition=off  SenseVelocity=off  SenseAcceleration=off  SenseTorqueForce=off  PositionTargetSpecify=on  PositionTargetPriority=Low  PositionTargetValue=2*Scissor_Lift_Param.Crossbar.Init_Angle_Target  PositionTargetValueUnits=deg  VelocityTargetSpecify=off  VelocityTargetPriority=High  VelocityTargetValue=0  VelocityTargetValueUnits=rad/s
  Rev RtIn : sm_lib/Joints/Revolute Joint  SenseConstraintForce=off  SenseConstraintForceX=off  SenseConstraintForceY=off  SenseConstraintForceZ=off  SenseConstraintTorque=off  SenseConstraintTorqueX=off  SenseConstraintTorqueY=off  SenseConstraintTorqueZ=off  SenseTotalForce=off  SenseTotalForceX=off  SenseTotalForceY=off  SenseTotalForceZ=off  SenseTotalTorque=off  SenseTotalTorqueX=off  SenseTotalTorqueY=off  SenseTotalTorqueZ=off  CompositeWrenchDir=FollowerOnBase  CompositeWrenchFrame=BaseFrame  EquilibriumPosition=0  EquilibriumPositionUnits=rad  SpringStiffness=0  SpringStiffnessUnits=N*m/rad  DampingCoefficient=0  DampingCoefficientUnits=N*m/(rad/s)  TorqueActuationMode=NoTorque  MotionActuationMode=ComputedMotion  SensePosition=off  SenseVelocity=off  SenseAcceleration=off  SenseTorqueForce=off  PositionTargetSpecify=off  PositionTargetPriority=Low  PositionTargetValue=0  PositionTargetValueUnits=deg  VelocityTargetSpecify=off  VelocityTargetPriority=High  VelocityTargetValue=0  VelocityTargetValueUnits=rad/s
  Rev RtOut : sm_lib/Joints/Revolute Joint  SenseConstraintForce=off  SenseConstraintForceX=off  SenseConstraintForceY=off  SenseConstraintForceZ=off  SenseConstraintTorque=off  SenseConstraintTorqueX=off  SenseConstraintTorqueY=off  SenseConstraintTorqueZ=off  SenseTotalForce=off  SenseTotalForceX=off  SenseTotalForceY=off  SenseTotalForceZ=off  SenseTotalTorque=off  SenseTotalTorqueX=off  SenseTotalTorqueY=off  SenseTotalTorqueZ=off  CompositeWrenchDir=FollowerOnBase  CompositeWrenchFrame=BaseFrame  EquilibriumPosition=0  EquilibriumPositionUnits=rad  SpringStiffness=0  SpringStiffnessUnits=N*m/rad  DampingCoefficient=0  DampingCoefficientUnits=N*m/(rad/s)  TorqueActuationMode=NoTorque  MotionActuationMode=ComputedMotion  SensePosition=off  SenseVelocity=off  SenseAcceleration=off  SenseTorqueForce=off  PositionTargetSpecify=off  PositionTargetPriority=Low  PositionTargetValue=0  PositionTargetValueUnits=deg  VelocityTargetSpecify=off  VelocityTargetPriority=High  VelocityTargetValue=0  VelocityTargetValueUnits=rad/s
  X : PMIOPort  Port=1  Side=Left
  A : PMIOPort  Port=2  Side=Right
  RLO : PMIOPort  Port=3  Side=Left
  FLI : PMIOPort  Port=4  Side=Left
  FRI : PMIOPort  Port=5  Side=Left
  RRO : PMIOPort  Port=6  Side=Left
  LO : PMIOPort  Port=7  Side=Right
  LI : PMIOPort  Port=8  Side=Right
  RI : PMIOPort  Port=9  Side=Right
  RO : PMIOPort  Port=10  Side=Right
  connections:
  X/RConn1 -- Bracket/LConn1 -- A/RConn1
  RO/RConn1 -- Rev RtOut/LConn1
  RI/RConn1 -- Rev RtIn/LConn1
  LO/RConn1 -- Rev LfOut/LConn1
  LI/RConn1 -- Rev LfIn/LConn1
  Rev RtOut/RConn1 -- RX/RConn2
  Rev RtIn/RConn1 -- RX/RConn1 -- Bracket/RConn2
  RX/LConn1 -- RShaft/RConn2
  RShaft/RConn1 -- RRO/RConn1
  RShaft/LConn1 -- RLO/RConn1
  Rev LfIn/RConn1 -- LX/RConn2 -- Bracket/RConn1
  Rev LfOut/RConn1 -- LX/RConn1
  LX/LConn2 -- RShaft/LConn2
  FShaft/RConn2 -- FRI/RConn1
  FShaft/RConn1 -- RX/LConn2
  FShaft/LConn2 -- FLI/RConn1
  FShaft/LConn1 -- LX/LConn1

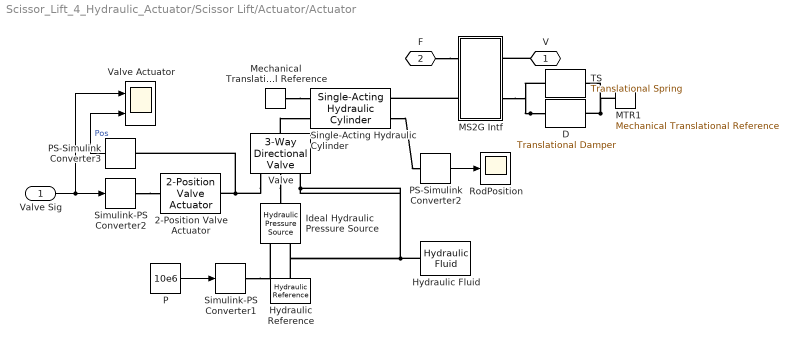
== system Scissor_Lift_4_Hydraulic_Actuator/Scissor Lift/Actuator/Actuator ==
  Valve Sig : Inport
  2-Position Valve Actuator : sh_lib/Valves/Valve Actuators/2-Position Valve Actuator  Tag=Factory Generic  stroke=0.01 m  t_on=0.1 s  t_off=0.1 s  act_signal=24  init_position=0  act_orientation=1
  D : fl_lib/Mechanical/Translational Elements/Translational Damper  Tag=Factory Generic  D=250+1000 N/(m/s)  v_specify=off  v_priority=High  v=0 m/s  f_specify=off  f_priority=High  f=0 N
  Hydraulic Fluid : sh_lib/Hydraulic Utilities/Hydraulic Fluid  Tag=Factory Generic  DataSource=1  SelFluid=1  SysTemp=40 c  TrapAir=0.002  ViscDerFactor=1  range_error=2
  Hydraulic Reference : fl_lib/Hydraulic/Hydraulic Elements/Hydraulic Reference  Tag=Factory Generic
  Ideal Hydraulic Pressure Source : fl_lib/Hydraulic/Hydraulic Sources/Hydraulic Pressure Source  Tag=Factory Generic
  MS2G Intf : Subsystem
  MTR1 : fl_lib/Mechanical/Translational Elements/Mechanical Translational Reference  Tag=Factory Generic
  Mechanical Translational Reference : fl_lib/Mechanical/Translational Elements/Mechanical Translational Reference  Tag=Factory Generic
  P : Constant  Value=10e6
  PS-Simulink Converter2 : nesl_utility/PS-Simulink Converter  PhysicalDomain=network_engine_domain  SubClassName=ps_output  LeftPortType=input  RightPortType=output  PseudoPeriodic=off  Frequencies=[]  Unit=1  AffineConversion=off
  PS-Simulink Converter3 : nesl_utility/PS-Simulink Converter  PhysicalDomain=network_engine_domain  SubClassName=ps_output  LeftPortType=input  RightPortType=output  PseudoPeriodic=off  Frequencies=[]  Unit=1  AffineConversion=off
  RodPosition : Scope
  Simulink-PS Converter1 : nesl_utility/Simulink-PS Converter  PhysicalDomain=network_engine_domain  SubClassName=ps_input  LeftPortType=input  RightPortType=output  PseudoPeriodic=off  Frequencies=[]  NoiseDistribution=none  NoiseParameters=[]  Unit=1  AffineConversion=off  InputFiltering=off  SimscapeFilterOrder=1  InputFilterTimeConstant=.001  UdotUserProvided=0
  Simulink-PS Converter2 : nesl_utility/Simulink-PS Converter  PhysicalDomain=network_engine_domain  SubClassName=ps_input  LeftPortType=input  RightPortType=output  PseudoPeriodic=off  Frequencies=[]  NoiseDistribution=none  NoiseParameters=[]  Unit=1  AffineConversion=off  InputFiltering=off  SimscapeFilterOrder=1  InputFilterTimeConstant=.001  UdotUserProvided=0
  Single-Acting Hydraulic Cylinder : sh_lib/Hydraulic Cylinders/Single-Acting Hydraulic Cylinder  Tag=Factory Generic  area=0.002 m^2  stroke=0.25*6 m  init_pos=0.05 m  dead_vol=1e-06 m^3  init_pressure=5e6 Pa  k_sh=1.4  stiff=1e+07 N/m  D=250 N/(m/s)  or=2
  TS : fl_lib/Mechanical/Translational Elements/Translational Spring  Tag=Factory Generic  spr_rate=6e3 N/m  v_specify=off  v_priority=High  v=0 m/s  f_specify=off  f_priority=High  f=0 N  x_specify=on  x_priority=High  x=0.02*0 m
  Valve : sh_lib/Valves/Directional Valves/3-Way Directional Valve  Tag=Factory Generic  mdl_type=1  area_max=1e-4*6 m^2  opening_max=0.01 m  opening_tab="[  -0.002 0 0.005 0.015 ] m"  area_tab="[  1e-12 4e-12 1e-05 1.02e-05 ] m^2"  pressure_tab="[  -5e+06 -2e+06 2e+06 5e+06 ] Pa"  flow_rate_tab="[  -1e-12 -6e-14 6e+12 1e+11 ; -8e-08 -4e-08 4e+06 8e+06 ; -0.0025 -0.00103 0.001 0.0024 ; -0.00258 -0.001032 0.00106 0.00247 ; ] m^3/s"  interp_method=1  extrap_method=1  C_d=0.7  x_0_P=0 m  x_0_T=-0.08 m  Re_cr=12  A_leak=1e-9 m^2
  Valve Actuator : Scope  NumInputPorts=2
  V : PMIOPort  Port=1  Side=Right
  F : PMIOPort  Port=2  Side=Left
  wires:
  P/1 -> Simulink-PS Converter1/1
  PS-Simulink Converter2/1 -> RodPosition/1
  PS-Simulink Converter3/1 -> Valve Actuator/2  "Pos"
  Valve Sig/1 -> Simulink-PS Converter2/1, Valve Actuator/1
  connections:
  Simulink-PS Converter2/RConn1 -- 2-Position Valve Actuator/LConn1
  2-Position Valve Actuator/RConn1 -- Valve/RConn1 -- PS-Simulink Converter3/LConn1
  Valve/LConn1 -- Single-Acting Hydraulic Cylinder/LConn2
  Valve/RConn2 -- Ideal Hydraulic Pressure Source/LConn1
  Valve/RConn3 -- Ideal Hydraulic Pressure Source/RConn2 -- Hydraulic Reference/LConn1 -- Hydraulic Fluid/RConn1
  D/LConn1 -- TS/LConn1 -- MS2G Intf/LConn2
  D/RConn1 -- MTR1/LConn1 -- TS/RConn1
  Simulink-PS Converter1/RConn1 -- Ideal Hydraulic Pressure Source/RConn1
  MS2G Intf/RConn2 -- Single-Acting Hydraulic Cylinder/RConn1
  Mechanical Translational Reference/LConn1 -- Single-Acting Hydraulic Cylinder/LConn1
  Single-Acting Hydraulic Cylinder/RConn2 -- PS-Simulink Converter2/LConn1
  V/RConn1 -- MS2G Intf/LConn1
  F/RConn1 -- MS2G Intf/RConn1
